simulink model "Delay"  (Simulink 8.3)
settings: Solver=FixedStepDiscrete  StartTime=0.0  StopTime=20  MaxStep=.2  RelTol=1e-3
libraries: dspsrcs4 x1, dspsigops x1
settings Model: Creator=Clay  LastModifiedBy=brks9622
settings OptimizationCC: ExpressionDepthLimit=2147483647
settings DebuggingCC: FcnCallInpInsideContextMsg=EnableAllAsWarning
settings HardwareCC: ProdBitPerChar=16  ProdBitPerInt=16  ProdBitPerPointer=16  ProdLargestAtomicInteger=Integer  ProdIntDivRoundTo=Zero  ProdEndianess=LittleEndian  ProdWordSize=16  ProdHWDeviceType=Texas Instruments->C2000
settings RTWCC: GenCodeOnly=on  BuildConfiguration=Faster Runs
settings GRTTargetCC: CombineOutputUpdateFcns=on  GRTInterface=off

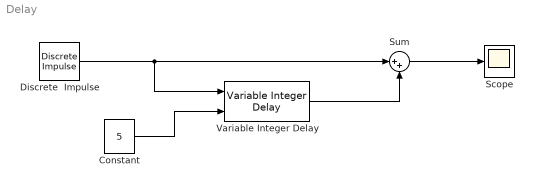
== system Delay ==
  Constant : Constant  Value=5  VectorParams1D=off
  Discrete  Impulse : dspsrcs4/Discrete  Impulse  Delay=2  SampleTime=1  FrameSample=1  dataType=double  isSigned=on  wordLen=16  udDataType=sfix(16)  fracBitsMode=Best precision  numFracBits=15  OutDataTypeStr=double  LastOutDataTypeStr=double
  Scope : Scope
  Sum : Sum  Inputs=|++
  Variable Integer Delay : dspsigops/Variable Integer Delay  dmax=22000  InputProcessing=Columns as channels (frame based)  ic=0  noDFT=off
  wires:
  Discrete  Impulse/1 -> Sum/1, Variable Integer Delay/1
  Variable Integer Delay/1 -> Sum/2
  Sum/1 -> Scope/1
  Constant/1 -> Variable Integer Delay/2
